simulink model "roverPlanPath_hw"  (R2020a)
settings: Solver=FixedStepAuto  StartTime=0.0  StopTime=100  FixedStep=TS  RelTol=1e-3  EnableMultiTasking=on
PostLoadFcn:
  | params
  | load('motorResponse.mat')
model workspace (MAT data in the model file):
  TS = 0.01
undefined symbols (not defined in the file): L, PWMcmdMono_L, PWMcmdMono_R, r, speedMono_L, speedMono_R, StartTheta
libraries: arduinomotorcarrierlib x4, simulink_extras x4, simulink x2
settings Model: SimulationMode=external  SILPILModeSetting=veronly  ExtModeTrigDuration=2  Creator=jmodiset  LastModifiedBy=mmarathe
settings DataIOCC: ReturnWorkspaceOutputs=off
settings OptimizationCC: PassReuseOutputArgsThreshold=0  MaxStackSize=64
settings DebuggingCC: UnderspecifiedInitializationDetection=Classic  MergeDetectMultiDrivingBlocksExec=none  ParameterTunabilityLossMsg=error  PregeneratedLibrarySubsystemCodeDiagnostic=none  ArithmeticOperatorsInVariantConditions=warning
settings HardwareCC: ProdBitPerPointer=32  ProdBitPerSizeT=32  ProdBitPerPtrDiffT=32  ProdLargestAtomicInteger=Long  ProdLargestAtomicFloat=Double  ProdWordSize=32  ProdHWDeviceType=ARM Compatible->ARM Cortex
settings SFSimCC: SimUseLocalCustomCode=off  MATLABDynamicMemAlloc=off  CustomCodeUndefinedFunction=UseInterfaceOnly
settings RTWCC: SystemTargetFile=ert.tlc  HardwareBoard=Arduino Nano 33 IoT  TLCOptions=-aInlineSetEventsForThisBaseRateFcn=TLC_FALSE -aSuppressMultiTaskScheduler=TLC_FALSE -aRateBasedStepFcn=1  TemplateMakefile=ert_default_tmf  RTWUseLocalCustomCode=off  Toolchain=Arduino ARM  BuildConfiguration=Faster Runs
settings CodeAppCC: ForceParamTrailComments=on  OperatorAnnotations=on
settings ERTTargetCC: ERTCustomFileBanners=off  SupportContinuousTime=on  SupportNonInlinedSFcns=on  RemoveResetFunc=off  SupportVariableSizeSignals=on  ModelStepFunctionPrototypeControlCompliant=off  ExtModeStaticAllocSize=8192

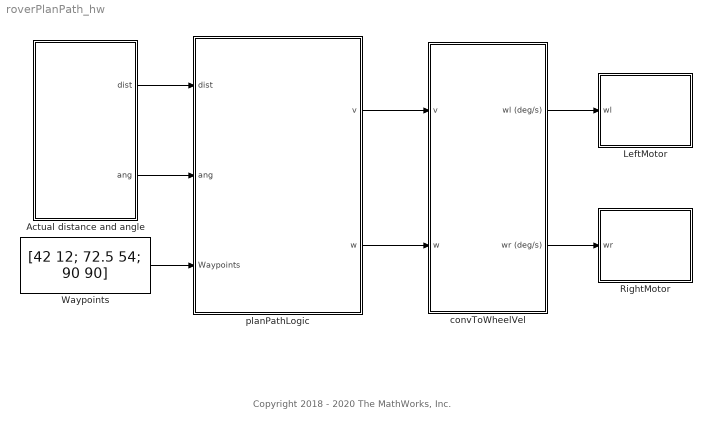
== system roverPlanPath_hw ==
  note: Copyright 2018 - 2020 The MathWorks, Inc.
  Actual distance and angle : Subsystem
  LeftMotor : Subsystem
      mask Display:
      | color('white');
      | plot([100,100,100,100]*1,[100,100,100,100]*1);
      | plot([100,100,100,100]*0,[100,100,100,100]*0);
      | sppkgroot = strrep(codertarget.arduinobase.internal.getBaseSpPkgRootDir(),'\','/');
      | image(fullfile(sppkgroot,'resources','dcmotor.png'),'center')
  RightMotor : Subsystem
      mask Display:
      | color('white');
      | plot([100,100,100,100]*1,[100,100,100,100]*1);
      | plot([100,100,100,100]*0,[100,100,100,100]*0);
      | sppkgroot = strrep(codertarget.arduinobase.internal.getBaseSpPkgRootDir(),'\','/');
      | image(fullfile(sppkgroot,'resources','dcmotor.png'),'center')
  Waypoints : Constant  Value=[42 12; 72.5 54; 90 90]
  convToWheelVel : Subsystem
  planPathLogic : Stateflow chart  TreatAsAtomicUnit=on
  wires:
  planPathLogic/2(w) -> convToWheelVel/2(w)
  planPathLogic/1(v) -> convToWheelVel/1(v)
  Actual distance and angle/1(dist) -> planPathLogic/1(dist)
  Actual distance and angle/2(ang) -> planPathLogic/2(ang)
  Waypoints/1 -> planPathLogic/3(Waypoints)
  convToWheelVel/1(wl (deg/s)) -> LeftMotor/1(wl)
  convToWheelVel/2(wr (deg/s)) -> RightMotor/1(wr)

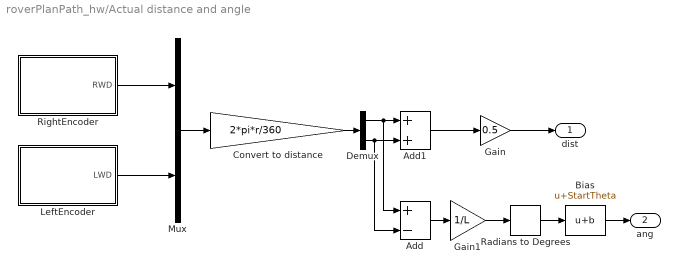
== system roverPlanPath_hw/Actual distance and angle ==
  Add : Sum  Inputs=+-
  Add1 : Sum
  Bias : Bias  Bias=StartTheta
  Convert to distance : Gain  Gain=2*pi*r/360
  Demux : Demux  Outputs=2
  Gain : Gain  Gain=0.5
  Gain1 : Gain  Gain=1/L
  LeftEncoder : Subsystem
  Mux : Mux  Inputs=2
  Radians to Degrees : simulink_extras/Transformations/Radians to Degrees
  RightEncoder : Subsystem
  dist : Outport  VectorParamsAs1DForOutWhenUnconnected=off
  ang : Outport  Port=2  VectorParamsAs1DForOutWhenUnconnected=off
  wires:
  RightEncoder/1(RWD) -> Mux/1
  Gain1/1 -> Radians to Degrees/1
  Add/1 -> Gain1/1
  Demux/2 -> Add1/2, Add/2
  Convert to distance/1 -> Demux/1
  Demux/1 -> Add1/1, Add/1
  Mux/1 -> Convert to distance/1
  LeftEncoder/1(LWD) -> Mux/2
  Radians to Degrees/1 -> Bias/1
  Add1/1 -> Gain/1
  Gain/1 -> dist/1
  Bias/1 -> ang/1

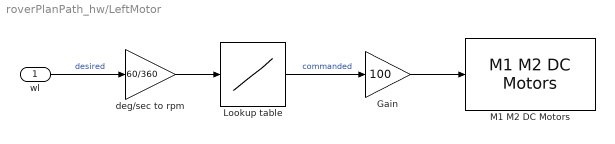
== system roverPlanPath_hw/LeftMotor ==
  wl : Inport
  Gain : Gain  Gain=100
  Lookup table : Lookup_n-D  NumberOfTableDimensions=1  BreakpointsForDimension1=speedMono_L  Table=PWMcmdMono_L  UseLastTableValue=on  InternalRulePriority=Speed  RndMeth=Simplest  InputSameDT=on
  M1 M2 DC Motors : arduinomotorcarrierlib/M1 M2 DC Motors  SlaveAddress=uint8( hex2dec( '66' ) )  blockPlatform=ARDUINO  MotorNumber=M2  MotorCarrierPWMFreq=100
      settings: SourceProductName=Simulink Support Package for Arduino Hardware
  deg/sec to rpm : Gain  Gain=60/360
  wires:
  wl/1 -> deg/sec to rpm/1  "desired"
  Lookup table/1 -> Gain/1  "commanded"
  Gain/1 -> M1 M2 DC Motors/1
  deg/sec to rpm/1 -> Lookup table/1

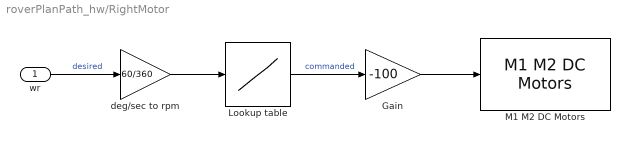
== system roverPlanPath_hw/RightMotor ==
  wr : Inport
  Gain : Gain  Gain=-100
  Lookup table : Lookup_n-D  NumberOfTableDimensions=1  BreakpointsForDimension1=speedMono_R  Table=PWMcmdMono_R  UseLastTableValue=on  InternalRulePriority=Speed  RndMeth=Simplest  InputSameDT=on
  M1 M2 DC Motors : arduinomotorcarrierlib/M1 M2 DC Motors  SlaveAddress=uint8( hex2dec( '66' ) )  blockPlatform=ARDUINO  MotorNumber=M1  MotorCarrierPWMFreq=100
      settings: SourceProductName=Simulink Support Package for Arduino Hardware
  deg/sec to rpm : Gain  Gain=60/360
  wires:
  wr/1 -> deg/sec to rpm/1  "desired"
  Lookup table/1 -> Gain/1  "commanded"
  Gain/1 -> M1 M2 DC Motors/1
  deg/sec to rpm/1 -> Lookup table/1

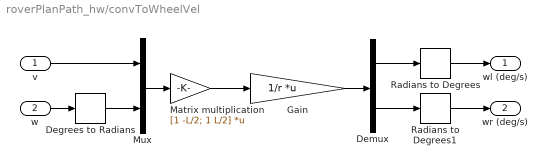
== system roverPlanPath_hw/convToWheelVel ==
  v : Inport
  w : Inport  Port=2
  " Gain" : Gain  Gain=1/r  Multiplication=Matrix(K*u)
  Degrees to Radians : simulink_extras/Transformations/Degrees to Radians
  Demux : Demux  Outputs=2
  Matrix multiplication : Gain  Gain=[1 -L/2; 1 L/2]  Multiplication=Matrix(K*u)
  Mux : Mux  Inputs=2
  Radians to Degrees : simulink_extras/Transformations/Radians to Degrees
  Radians to Degrees1 : simulink_extras/Transformations/Radians to Degrees
  wl (deg/s) : Outport  VectorParamsAs1DForOutWhenUnconnected=off
  wr (deg/s) : Outport  Port=2  VectorParamsAs1DForOutWhenUnconnected=off
  wires:
  " Gain"/1 -> Demux/1
  Matrix multiplication/1 -> " Gain"/1
  v/1 -> Mux/1
  Mux/1 -> Matrix multiplication/1
  Demux/1 -> Radians to Degrees/1
  Demux/2 -> Radians to Degrees1/1
  w/1 -> Degrees to Radians/1
  Radians to Degrees/1 -> wl (deg/s)/1
  Radians to Degrees1/1 -> wr (deg/s)/1
  Degrees to Radians/1 -> Mux/2

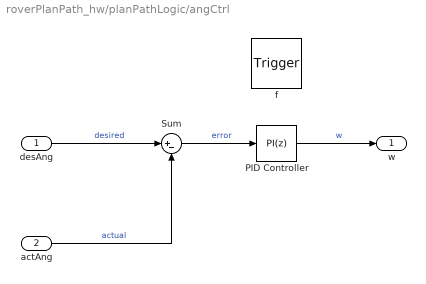
== system roverPlanPath_hw/planPathLogic/angCtrl ==
  desAng : Inport  OutDataTypeStr=double  PortDimensions=1
  actAng : Inport  Port=2  OutDataTypeStr=double  PortDimensions=1
  f : TriggerPort  TriggerType=function-call  VariantControl=(inherit)
      settings: CopyFcn=Stateflow.SLINSF.SimulinkMan.removeBlockPreDeleteFcn  PreDeleteFcn=Stateflow.SLINSF.SimulinkMan.unsafePredeleteFcn
  PID Controller : simulink/Continuous/PID Controller  Controller=PI  Form=Parallel  TimeDomain=Discrete-time  UseExternalTs=off  SampleTime=-1  IntegratorMethod=Forward Euler  FilterMethod=Forward Euler  ControllerParametersSource=internal  P=3  I=1  D=0  UseFilter=on  N=100  TunerSelectOption=Transfer Function Based (PID Tuner App)  InitialConditionSource=internal  InitialConditionForIntegrator=0  InitialConditionForFilter=0  DifferentiatorICPrevScaledInput=0  ExternalReset=none  TrackingMode=off  Kt=1  LimitOutput=off  UpperSaturationLimit=inf  LowerSaturationLimit=-inf  LinearizeAsGain=on  AntiWindupMode=none  Kb=1  POutMin=[]  POutMax=[]  IOutMin=[]  IOutMax=[]  DOutMin=[]  DOutMax=[]  NOutMin=[]  NOutMax=[]  SumOutMin=[]  SumOutMax=[]  SaturationOutMin=[]  SaturationOutMax=[]  PParamMin=[]  PParamMax=[]  IParamMin=[]  IParamMax=[]  DParamMin=[]  DParamMax=[]  NParamMin=[]  NParamMax=[]  KbParamMin=[]  KbParamMax=[]  KtParamMin=[]  KtParamMax=[]  KbOutMin=[]  KbOutMax=[]  KtOutMin=[]  KtOutMax=[]  IntegratorOutMin=[]  IntegratorOutMax=[]  FilterOutMin=[]  FilterOutMax=[]  SumI1OutMin=[]  SumI1OutMax=[]  SumI2OutMin=[]  SumI2OutMax=[]  SumI3OutMin=[]  SumI3OutMax=[]  SumI4OutMin=[]  SumI4OutMax=[]  SumDOutMin=[]  SumDOutMax=[]  DifferentiatorOutMin=[]  DifferentiatorOutMax=[]  FilterDiffOutCoefMin=[]  FilterDiffOutCoefMax=[]  ReciprocalOutMin=[]  ReciprocalOutMax=[]  SumDenOutMin=[]  SumDenOutMax=[]  SumNumOutMin=[]  SumNumOutMax=[]  DivideOutMin=[]  DivideOutMax=[]  UdiffTsProdOutMin=[]  UdiffTsProdOutMax=[]  NTsProdOutMin=[]  NTsProdOutMax=[]  UintegralTsProdOutMin=[]  UintegralTsProdOutMax=[]  UngainTsProdOutMin=[]  UngainTsProdOutMax=[]  IntegratorContinuousStateAttributes=''  IntegratorStateMustResolveToSignalObject=off  IntegratorRTWStateStorageClass=Auto  FilterContinuousStateAttributes=''  FilterStateMustResolveToSignalObject=off  FilterRTWStateStorageClass=Auto  ParallelPVariant=InternalParameters  IdealPVariant=Disabled  IVariant=InternalParameters  DVariant=Disabled  IntegratorVariant=Discrete  SatVariant=Disabled  AWVariant=Passthrough  PCopyVariant=Disabled  TRVariant=Disabled  FdbkBlocksVariant=Forward  IdealPFdbkVariant=Disabled  SatFdbkVariant=Disabled  DerivativeFilterVariant=Disabled  NVariant=Disabled  NCopyVariant=Disabled_SignalSpec  FilterICVariant=Disabled  IntegratorICVariant=InternalICs  ExternalResetVariant=Disabled  TRSumVariant=Passthrough  SumFdbkVariant=Disabled  SumVariant=Sum_PI  TsampFilterVariant=InternalTs  TsampNgainVariant=Passthrough  TsampIntegralVariant=Passthrough
  Sum : Sum  Inputs=|+-
  w : Outport  VectorParamsAs1DForOutWhenUnconnected=off
  wires:
  actAng/1 -> Sum/2  "actual"
  desAng/1 -> Sum/1  "desired"
  PID Controller/1 -> w/1  "w"
  Sum/1 -> PID Controller/1  "error"

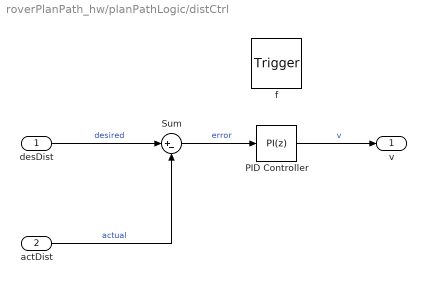
== system roverPlanPath_hw/planPathLogic/distCtrl ==
  desDist : Inport  OutDataTypeStr=double  PortDimensions=1
  actDist : Inport  Port=2  OutDataTypeStr=double  PortDimensions=1
  f : TriggerPort  TriggerType=function-call  VariantControl=(inherit)
      settings: CopyFcn=Stateflow.SLINSF.SimulinkMan.removeBlockPreDeleteFcn  PreDeleteFcn=Stateflow.SLINSF.SimulinkMan.unsafePredeleteFcn
  PID Controller : simulink/Continuous/PID Controller  Controller=PI  Form=Parallel  TimeDomain=Discrete-time  UseExternalTs=off  SampleTime=-1  IntegratorMethod=Forward Euler  FilterMethod=Forward Euler  ControllerParametersSource=internal  P=0.2  I=0.001  D=0  UseFilter=on  N=100  TunerSelectOption=Transfer Function Based (PID Tuner App)  InitialConditionSource=internal  InitialConditionForIntegrator=0  InitialConditionForFilter=0  DifferentiatorICPrevScaledInput=0  ExternalReset=none  TrackingMode=off  Kt=1  LimitOutput=off  UpperSaturationLimit=inf  LowerSaturationLimit=-inf  LinearizeAsGain=on  AntiWindupMode=none  Kb=1  POutMin=[]  POutMax=[]  IOutMin=[]  IOutMax=[]  DOutMin=[]  DOutMax=[]  NOutMin=[]  NOutMax=[]  SumOutMin=[]  SumOutMax=[]  SaturationOutMin=[]  SaturationOutMax=[]  PParamMin=[]  PParamMax=[]  IParamMin=[]  IParamMax=[]  DParamMin=[]  DParamMax=[]  NParamMin=[]  NParamMax=[]  KbParamMin=[]  KbParamMax=[]  KtParamMin=[]  KtParamMax=[]  KbOutMin=[]  KbOutMax=[]  KtOutMin=[]  KtOutMax=[]  IntegratorOutMin=[]  IntegratorOutMax=[]  FilterOutMin=[]  FilterOutMax=[]  SumI1OutMin=[]  SumI1OutMax=[]  SumI2OutMin=[]  SumI2OutMax=[]  SumI3OutMin=[]  SumI3OutMax=[]  SumI4OutMin=[]  SumI4OutMax=[]  SumDOutMin=[]  SumDOutMax=[]  DifferentiatorOutMin=[]  DifferentiatorOutMax=[]  FilterDiffOutCoefMin=[]  FilterDiffOutCoefMax=[]  ReciprocalOutMin=[]  ReciprocalOutMax=[]  SumDenOutMin=[]  SumDenOutMax=[]  SumNumOutMin=[]  SumNumOutMax=[]  DivideOutMin=[]  DivideOutMax=[]  UdiffTsProdOutMin=[]  UdiffTsProdOutMax=[]  NTsProdOutMin=[]  NTsProdOutMax=[]  UintegralTsProdOutMin=[]  UintegralTsProdOutMax=[]  UngainTsProdOutMin=[]  UngainTsProdOutMax=[]  IntegratorContinuousStateAttributes=''  IntegratorStateMustResolveToSignalObject=off  IntegratorRTWStateStorageClass=Auto  FilterContinuousStateAttributes=''  FilterStateMustResolveToSignalObject=off  FilterRTWStateStorageClass=Auto  ParallelPVariant=InternalParameters  IdealPVariant=Disabled  IVariant=InternalParameters  DVariant=Disabled  IntegratorVariant=Discrete  SatVariant=Disabled  AWVariant=Passthrough  PCopyVariant=Disabled  TRVariant=Disabled  FdbkBlocksVariant=Forward  IdealPFdbkVariant=Disabled  SatFdbkVariant=Disabled  DerivativeFilterVariant=Disabled  NVariant=Disabled  NCopyVariant=Disabled_SignalSpec  FilterICVariant=Disabled  IntegratorICVariant=InternalICs  ExternalResetVariant=Disabled  TRSumVariant=Passthrough  SumFdbkVariant=Disabled  SumVariant=Sum_PI  TsampFilterVariant=InternalTs  TsampNgainVariant=Passthrough  TsampIntegralVariant=Passthrough
  Sum : Sum  Inputs=|+-
  v : Outport  VectorParamsAs1DForOutWhenUnconnected=off
  wires:
  actDist/1 -> Sum/2  "actual"
  desDist/1 -> Sum/1  "desired"
  PID Controller/1 -> v/1  "v"
  Sum/1 -> PID Controller/1  "error"

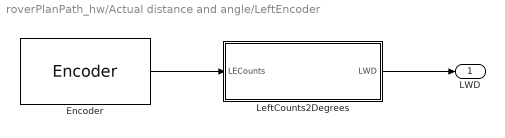
== system roverPlanPath_hw/Actual distance and angle/LeftEncoder ==
  Encoder : arduinomotorcarrierlib/Encoder  SlaveAddress=uint8( hex2dec( '66' ) )  blockPlatform=ARDUINO  Encoder=2  ShowSpeed=off  ResetOption=on  SampleTime=0.01
      settings: SourceProductBaseCode=ARDUINO
  LeftCounts2Degrees : Subsystem
  LWD : Outport  VectorParamsAs1DForOutWhenUnconnected=off
  wires:
  LeftCounts2Degrees/1(LWD) -> LWD/1
  Encoder/1 -> LeftCounts2Degrees/1(LECounts)

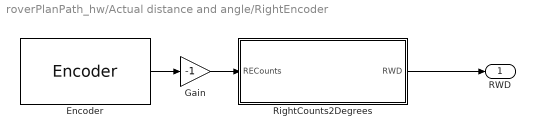
== system roverPlanPath_hw/Actual distance and angle/RightEncoder ==
  Encoder : arduinomotorcarrierlib/Encoder  SlaveAddress=uint8( hex2dec( '66' ) )  blockPlatform=ARDUINO  Encoder=1  ShowSpeed=off  ResetOption=on  SampleTime=0.01
      settings: SourceProductBaseCode=ARDUINO
  Gain : Gain  Gain=-1
  RightCounts2Degrees : Subsystem
  RWD : Outport  VectorParamsAs1DForOutWhenUnconnected=off
  wires:
  RightCounts2Degrees/1(RWD) -> RWD/1
  Encoder/1 -> Gain/1
  Gain/1 -> RightCounts2Degrees/1(RECounts)

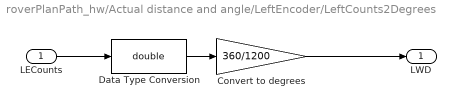
== system roverPlanPath_hw/Actual distance and angle/LeftEncoder/LeftCounts2Degrees ==
  LECounts : Inport
  Convert to degrees : Gain  Gain=360/1200
  Data Type Conversion : DataTypeConversion  OutDataTypeStr=double
  LWD : Outport  VectorParamsAs1DForOutWhenUnconnected=off
  wires:
  LECounts/1 -> Data Type Conversion/1
  Data Type Conversion/1 -> Convert to degrees/1
  Convert to degrees/1 -> LWD/1

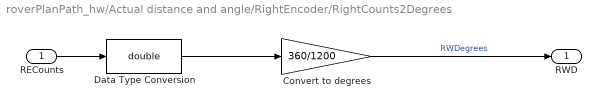
== system roverPlanPath_hw/Actual distance and angle/RightEncoder/RightCounts2Degrees ==
  RECounts : Inport
  Convert to degrees : Gain  Gain=360/1200
  Data Type Conversion : DataTypeConversion  OutDataTypeStr=double
  RWD : Outport  VectorParamsAs1DForOutWhenUnconnected=off
  wires:
  Data Type Conversion/1 -> Convert to degrees/1
  RECounts/1 -> Data Type Conversion/1
  Convert to degrees/1 -> RWD/1  "RWDegrees"

== stateflow chart roverPlanPath_hw/planPathLogic ==
  state Pause
    entry:
    v = 0; w= 0;
  state Turn
    entry:
    desAng = calcAngle(nextWPIndex);
    during, exit:
    v = 0;
    w = angCtrl(desAng,ang);
  state MoveForward
    entry:
    desDist = calcDist(nextWPIndex)+dist;
    during, exit:
    v = distCtrl(desDist, dist);
    w = 0;
  state w = angCtrl(desAng,actAng) [function]
  state v = distCtrl(desDist,actDist) [function]
  state Stop
    entry:
    v = 0;
    w = 0;
  (default) -> Pause
  Pause -> Turn : after(1,sec)
  Turn -> MoveForward : [abs(desAng - ang) < 1]
  MoveForward -> (junction 101) : [abs(desDist - dist) < 0.1]{nextWPIndex = nextWPIndex+1}
  (junction 101) -> Turn [order 2]
  (junction 101) -> Stop [order 1] : [nextWPIndex == size(Waypoints,1)]
  data: desAngle function_output; Index function_input; desDistance function_output; Index function_input; desAng function_input double size=1; actAng function_input double size=1; w function_output; desDist function_input double size=1; actDist function_input double size=1; v function_output; dist input; ang input; v output double size=1; w output double size=1; desDist local; desAng local; Waypoints input; nextWPIndex local =1
  function desAngle  = calcAngle(Index):
    | function desAngle  = calcAngle(Index)
    | 
    | toReachX = Waypoints(Index+1,1);
    | toReachY = Waypoints(Index+1,2);
    | x = Waypoints(Index,1);
    | y = Waypoints(Index,2);
    | distX = toReachX - x;
    | distY = toReachY - y;
    | if distX > 0 && distY >= 0
    |     quadrant = 1;
    | elseif distX <= 0 && distY > 0
    |     quadrant = 2;
    | elseif distX < 0 && distY <= 0
    |     quadrant = 3;
    | elseif distX >= 0 && distY < 0
    |     quadrant = 4;
    | else
    |     quadrant = 0;
    | end
    | desAngle = atand((toReachY-y)/(toReachX-x));
    | switch quadrant
    |     case 1
    |         
    |     case 2
    |         desAngle = 180-abs(desAngle);
    |     case 3
    |         desAngle = 180+desAngle;
    |     case 4
    |         desAngle = 360+desAngle;
    |     otherwise 
    |         desAngle = 0;
    | end
    | if desAngle > 360 
    |     desAngle = desAngle - 360;
    | end
    | end
  function desDistance = calcDist(Index):
    | function desDistance = calcDist(Index)
    | 
    | toReachX = Waypoints(Index+1,1);
    | toReachY = Waypoints(Index+1,2);
    | x = Waypoints(Index,1);
    | y = Waypoints(Index,2);
    | distX = toReachX - x;
    | distY = toReachY - y;
    | desDistance = sqrt(distX^2+distY^2);
    | end
